simulink model "HalfCar"  (R2020b)
settings: Solver=VariableStepAuto  StartTime=0.0  StopTime=2  MaxStep=0.0001  RelTol=1e-3
values from neighbouring files (symbols this model uses):
  a = 1.233    [main.m]
  Aobs = Aaug-L*Caug    [main.m]
  b = 1.327    [main.m]
  Bobs = [L, Baug]    [main.m]
  Cobs = eye(10)    [main.m]
  Dobs = zeros(10,6)    [main.m]
  kalmanFilter = ss(A_kalman,B_kalman,C_kalman,0)    [main.m]
  Kfeedback = struct('Kf',KFeedb(:,1:8),'P',P)    [main.m]
  KFeedbIntegratore = struct('Kfe',K(:,1:8),'Ki',K(:,9:10),'P',[P,-15-0.1i,-15+.1i ])    [main.m]
  KLQI = struct('KfeLQR',KLQInt(:,1:8),'KiLQR',KLQInt(:,9:10))    [main.m]
  KLQR = struct('KfeLQR',KLQ1(:,1:8))    [main.m]
  varIngressi = 150    [main.m]
  varPhi = 1.0000e-8    (= 1e-08)    [main.m]
  varPhiDot = 1.0000e-7    (= 1e-07)    [main.m]
  varZc = 1.0000e-8    (= 1e-08)    [main.m]
  varZcDot = 1.0000e-7    (= 1e-07)    [main.m]
  veicoloConDisturbi = ss(A,[B,L],C,0)    [main.m]
  vms = convvel(vkmh, 'km/h', 'm/s')    [main.m]
libraries: simulink_extras x18, simulink x2
settings Model: Creator=fadir  LastModifiedBy=fadir

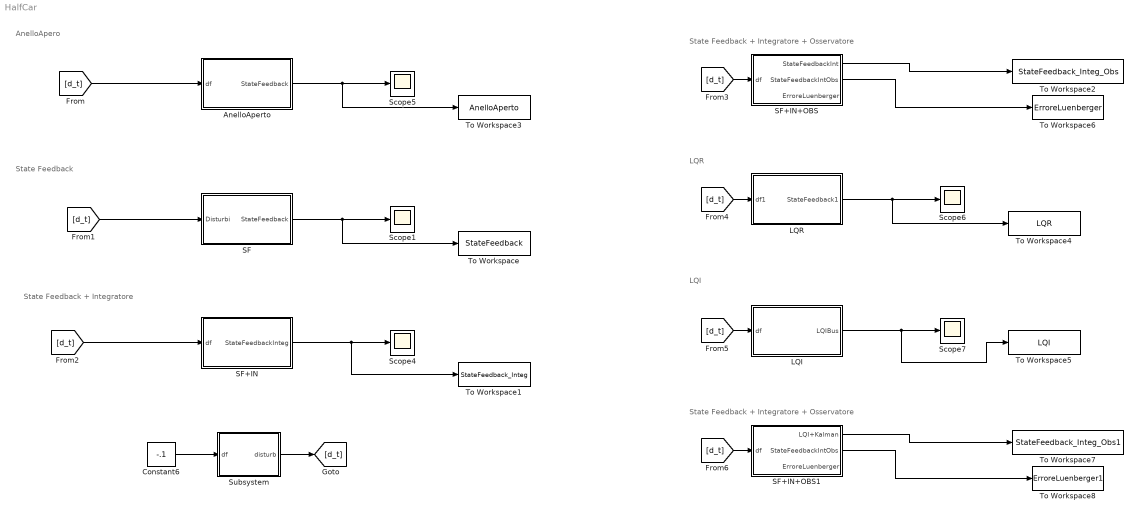
== system HalfCar ==
  note: State Feedback
  note: State Feedback + Integratore + Osservatore
  note: State Feedback + Integratore
  note: AnelloApero
  note: LQR
  note: LQI
  note: State Feedback + Integratore + Osservatore
  AnelloAperto : Subsystem
  Constant6 : Constant  Value=-.1
  LQI : Subsystem
  LQR : Subsystem
  SF : Subsystem
  SF+IN : Subsystem
  SF+IN+OBS : Subsystem
  SF+IN+OBS1 : Subsystem
  Scope{1,4..7} (5 alike) : Scope
  Subsystem : Subsystem
  To Workspace : ToWorkspace  VariableName=StateFeedback  SaveFormat=Timeseries  SampleTime=-1
  To Workspace1 : ToWorkspace  VariableName=StateFeedback_Integ  SaveFormat=Timeseries  SampleTime=-1
  To Workspace2 : ToWorkspace  VariableName=StateFeedback_Integ_Obs  SaveFormat=Timeseries  SampleTime=-1
  To Workspace3 : ToWorkspace  VariableName=AnelloAperto  SaveFormat=Timeseries  SampleTime=-1
  To Workspace4 : ToWorkspace  VariableName=LQR  SaveFormat=Timeseries  SampleTime=-1
  To Workspace5 : ToWorkspace  VariableName=LQI  SaveFormat=Timeseries  SampleTime=-1
  To Workspace6 : ToWorkspace  VariableName=ErroreLuenberger  SaveFormat=Timeseries  SampleTime=-1
  To Workspace7 : ToWorkspace  VariableName=StateFeedback_Integ_Obs1  SaveFormat=Timeseries  SampleTime=-1
  To Workspace8 : ToWorkspace  VariableName=ErroreLuenberger1  SaveFormat=Timeseries  SampleTime=-1
  wires:
  SF/1(StateFeedback) -> To Workspace/1, Scope1/1
  SF+IN+OBS/2(StateFeedbackIntObs) -> To Workspace6/1
  [d_t] -> SF/1(Disturbi)
  [d_t] -> SF+IN+OBS/1(df)
  [d_t] -> SF+IN/1(df)
  SF+IN/1(StateFeedbackInteg) -> To Workspace1/1, Scope4/1
  SF+IN+OBS/1(StateFeedbackInt) -> To Workspace2/1
  AnelloAperto/1(StateFeedback) -> To Workspace3/1, Scope5/1
  [d_t] -> AnelloAperto/1(df)
  [d_t] -> LQR/1(df1)
  LQR/1(StateFeedback1) -> Scope6/1, To Workspace4/1
  LQI/1(LQIBus) -> Scope7/1, To Workspace5/1
  [d_t] -> LQI/1(df)
  Constant6/1 -> Subsystem/1(df)
  Subsystem/1(" disturb") -> [d_t]
  SF+IN+OBS1/1(LQI+Kalman) -> To Workspace7/1
  [d_t] -> SF+IN+OBS1/1(df)
  SF+IN+OBS1/2(StateFeedbackIntObs) -> To Workspace8/1

== system HalfCar/AnelloAperto ==
  df : Inport
  Bus to Vector : BusToVector
  Mux : Mux  Inputs=[2 2]
  State-Space : StateSpace  A=veicoloConDisturbi.A  B=veicoloConDisturbi.B  C=eye(8)  D=zeros(8,4)  InitialCondition=0
  StateFeedbackBus : Subsystem
  StateFeedback : Outport
  wires:
  df/1 -> Bus to Vector/1
  State-Space/1 -> [x_real]  "states"
  Bus to Vector/1 -> Mux/2
  StateFeedbackBus/1(StateFeedback) -> StateFeedback/1
  Mux/1 -> State-Space/1
  [x_real] -> StateFeedbackBus/1(states)

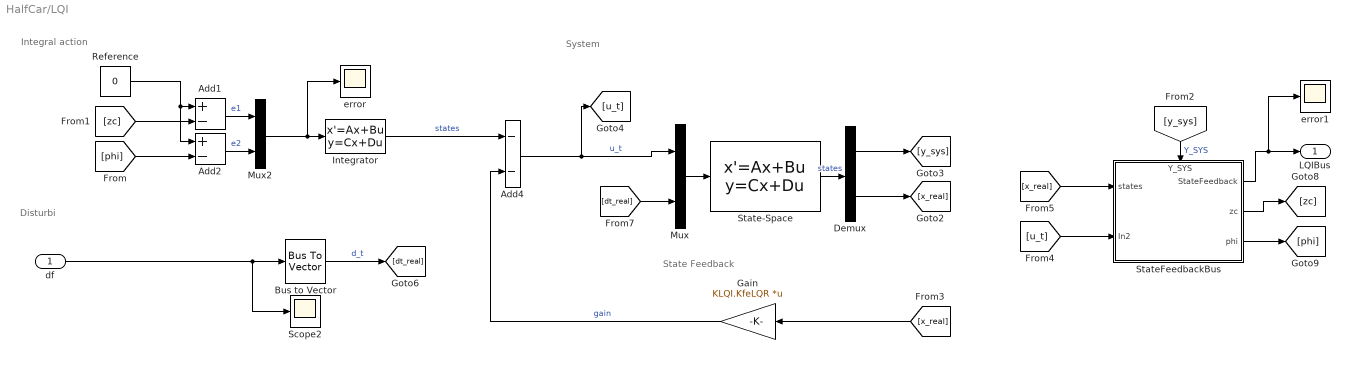
== system HalfCar/LQI ==
  note: System
  note: Integral action
  note: Disturbi
  note: State Feedback
  df : Inport
  Add1 : Sum  Inputs=+-
  Add2 : Sum  Inputs=+-
  Add4 : Sum  Inputs=--
  Bus to Vector : BusToVector
  Demux : Demux  Outputs=[4 8]
  Gain : Gain  Gain=KLQI.KfeLQR  Multiplication=Matrix(K*u)
  Integrator : StateSpace  A=zeros(2,2)  B=KLQI.KiLQR  C=eye(2)  D=zeros(2,2)  InitialCondition=0
  Mux : Mux  Inputs=[2 2]
  Mux2 : Mux  Inputs=2
  Reference : Constant  Value=0
  Scope2 : Scope
  State-Space : StateSpace  A=veicoloConDisturbi.A  B=veicoloConDisturbi.B  C=[veicoloConDisturbi.C;eye(8)]  D=zeros(12,4)  InitialCondition=0
  StateFeedbackBus : Subsystem
      settings: PortSchema="{\"entries\":[{\"content\":{\"sides\":[{\"content\":{\"connectorIds\":[\"In1\",\"In2\"]},\"type\":\"ConnectorPlacement.EquallySpacedRectSide\",\"uuid\":\"f033b987-6b3a-458c-bcac-b7c517520bbe\"},{\"content\":{\"connectorIds\":[\"Out1\",\"Out2\",\"Out3\"],\"side\":\"RIGHT\"},\"type\":\"ConnectorPlacement.EquallySpacedRectSide\",\"uuid\":\"ed7cee92-f0bc-4ba3-a5c5-3396d8293c14\"},{\"content\":{\"connectorIds\":[\"In3\"],\"side\":\"TOP\"},\"type\":\"ConnectorPlacement.EquallySpacedRectSide\",\"uuid\":\"4252f29c-7653-43d7-b93b-010ed3ee46e3\"},{\"content\":{\"connectorIds\":[],\"side\":\"HIDDEN\"},\"type\":\"ConnectorPlacement.EquallySpacedRectSide\",\"uuid\":\"adbffe9e-afd0-46bb-bf47-88a6e7d4714f\"}]},\"type\":\"ConnectorPlacement.EquallySpacedConnector\",\"uuid\":\"76cb68ad-0c01-48a8-b73c-8d6b8ab451c8\"}],\"packageUris\":[\"http://schema.mathworks.com/mf0/Connector/R2020b\"],\"version\":\"1.0\"}"
  error : Scope
  error1 : Scope
  LQIBus : Outport
  wires:
  StateFeedbackBus/2(zc) -> [zc]
  StateFeedbackBus/3(phi) -> [phi]
  StateFeedbackBus/1(" StateFeedback") -> error1/1, LQIBus/1
  [x_real] -> StateFeedbackBus/1(states)
  df/1 -> Bus to Vector/1, Scope2/1
  [zc] -> Add1/2
  [phi] -> Add2/2
  Bus to Vector/1 -> [dt_real]  "d_t"
  Add2/1 -> Mux2/2  "e2"
  Add1/1 -> Mux2/1  "e1"
  Reference/1 -> Add1/1, Add2/1
  Add4/1 -> [u_t], Mux/1  "u_t"
  Integrator/1 -> Add4/1  "states"
  Mux2/1 -> Integrator/1, error/1
  Gain/1 -> Add4/2  "gain"
  Mux/1 -> State-Space/1
  State-Space/1 -> Demux/1  "states"
  Demux/2 -> [x_real]
  [x_real] -> Gain/1
  Demux/1 -> [y_sys]
  [dt_real] -> Mux/2
  [u_t] -> StateFeedbackBus/2(In2)
  [y_sys] -> StateFeedbackBus/3(Y_SYS)  "Y_SYS"

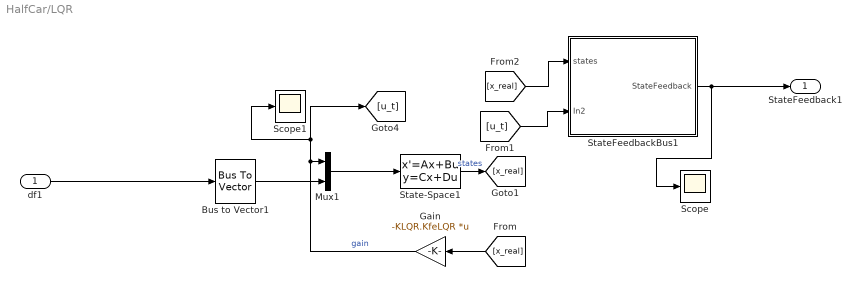
== system HalfCar/LQR ==
  df1 : Inport
  Bus to Vector1 : BusToVector
  Gain : Gain  Gain=-KLQR.KfeLQR  Multiplication=Matrix(K*u)
  Mux1 : Mux  Inputs=[2 2]
  Scope : Scope
  Scope1 : Scope
  State-Space1 : StateSpace  A=veicoloConDisturbi.A  B=veicoloConDisturbi.B  C=eye(8)  D=zeros(8,4)  InitialCondition=0
  StateFeedbackBus1 : Subsystem
  StateFeedback1 : Outport
  wires:
  Mux1/1 -> State-Space1/1
  df1/1 -> Bus to Vector1/1
  State-Space1/1 -> [x_real]  "states"
  Gain/1 -> [u_t], Scope1/1, Mux1/1  "gain"
  [x_real] -> StateFeedbackBus1/1(states)
  [x_real] -> Gain/1
  StateFeedbackBus1/1(StateFeedback) -> Scope/1, StateFeedback1/1
  Bus to Vector1/1 -> Mux1/2
  [u_t] -> StateFeedbackBus1/2(In2)

== system HalfCar/SF ==
  Disturbi : Inport
  Bus to Vector : BusToVector
  Gain : Gain  Gain=-1
  Mux : Mux  Inputs=[2 2]
  RetroazStato : Gain  Gain=Kfeedback.Kf  Multiplication=Matrix(K*u)
  Sistema : StateSpace  A=veicoloConDisturbi.A  B=veicoloConDisturbi.B  C=eye(8)  D=zeros(8,4)  InitialCondition=0
  StateFeedbackBus : Subsystem
  StateFeedback : Outport
  wires:
  RetroazStato/1 -> Gain/1  "gain"
  Disturbi/1 -> Bus to Vector/1
  Sistema/1 -> [x_real]  "states"
  Bus to Vector/1 -> Mux/2
  StateFeedbackBus/1(StateFeedback) -> StateFeedback/1
  Mux/1 -> Sistema/1
  [x_real] -> RetroazStato/1
  [x_real] -> StateFeedbackBus/2(states)
  [u_t] -> StateFeedbackBus/1(u_t)
  Gain/1 -> [u_t], Mux/1

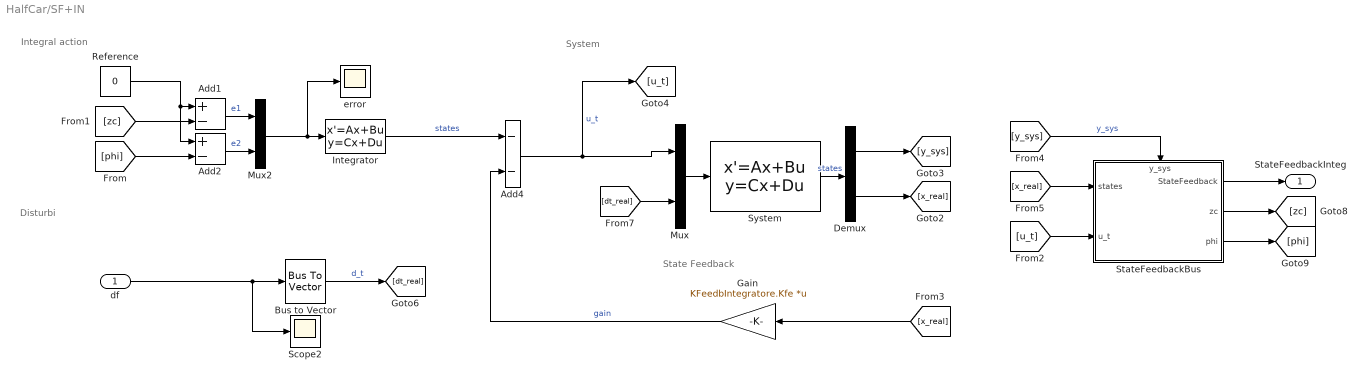
== system HalfCar/SF+IN ==
  note: State Feedback
  note: Disturbi
  note: Integral action
  note: System
  df : Inport
  Add1 : Sum  Inputs=+-
  Add2 : Sum  Inputs=+-
  Add4 : Sum  Inputs=--
  Bus to Vector : BusToVector
  Demux : Demux  Outputs=[4 8]
  Gain : Gain  Gain=KFeedbIntegratore.Kfe  Multiplication=Matrix(K*u)
  Integrator : StateSpace  A=zeros(2,2)  B=KFeedbIntegratore.Ki  C=eye(2)  D=zeros(2,2)  InitialCondition=0
  Mux : Mux  Inputs=[2 2]
  Mux2 : Mux  Inputs=2
  Reference : Constant  Value=0
  Scope2 : Scope
  StateFeedbackBus : Subsystem
      settings: PortSchema="{\"entries\":[{\"content\":{\"sides\":[{\"content\":{\"connectorIds\":[\"In1\",\"In2\"]},\"type\":\"ConnectorPlacement.EquallySpacedRectSide\",\"uuid\":\"7521623e-7228-4753-a009-bff90efec3f5\"},{\"content\":{\"connectorIds\":[\"Out1\",\"Out2\",\"Out3\"],\"side\":\"RIGHT\"},\"type\":\"ConnectorPlacement.EquallySpacedRectSide\",\"uuid\":\"ccf95793-c50d-4e88-afee-999bf5e64e87\"},{\"content\":{\"connectorIds\":[\"In3\"],\"side\":\"TOP\"},\"type\":\"ConnectorPlacement.EquallySpacedRectSide\",\"uuid\":\"63dab736-c292-47ee-a3b5-f2c1b3d06bd7\"},{\"content\":{\"connectorIds\":[],\"side\":\"HIDDEN\"},\"type\":\"ConnectorPlacement.EquallySpacedRectSide\",\"uuid\":\"ac2eb349-1c44-417c-9d28-b58d5fbdbdcb\"}]},\"type\":\"ConnectorPlacement.EquallySpacedConnector\",\"uuid\":\"e4851e5d-b044-4786-a828-79466b73b9fe\"}],\"packageUris\":[\"http://schema.mathworks.com/mf0/Connector/R2020b\"],\"version\":\"1.0\"}"
  System : StateSpace  A=veicoloConDisturbi.A  B=veicoloConDisturbi.B  C=[veicoloConDisturbi.C;eye(8)]  D=zeros(12,4)  InitialCondition=0
  error : Scope
  StateFeedbackInteg : Outport
  wires:
  [dt_real] -> Mux/2
  Demux/1 -> [y_sys]
  [x_real] -> Gain/1
  Demux/2 -> [x_real]
  System/1 -> Demux/1  "states"
  Mux/1 -> System/1
  Gain/1 -> Add4/2  "gain"
  Mux2/1 -> error/1, Integrator/1
  Integrator/1 -> Add4/1  "states"
  Add4/1 -> [u_t], Mux/1  "u_t"
  Reference/1 -> Add2/1, Add1/1
  Add1/1 -> Mux2/1  "e1"
  Add2/1 -> Mux2/2  "e2"
  Bus to Vector/1 -> [dt_real]  "d_t"
  [phi] -> Add2/2
  [zc] -> Add1/2
  df/1 -> Scope2/1, Bus to Vector/1
  [x_real] -> StateFeedbackBus/1(states)
  StateFeedbackBus/1(" StateFeedback") -> StateFeedbackInteg/1
  StateFeedbackBus/3(phi) -> [phi]
  StateFeedbackBus/2(zc) -> [zc]
  [u_t] -> StateFeedbackBus/2(u_t)
  [y_sys] -> StateFeedbackBus/3(y_sys)  "y_sys"

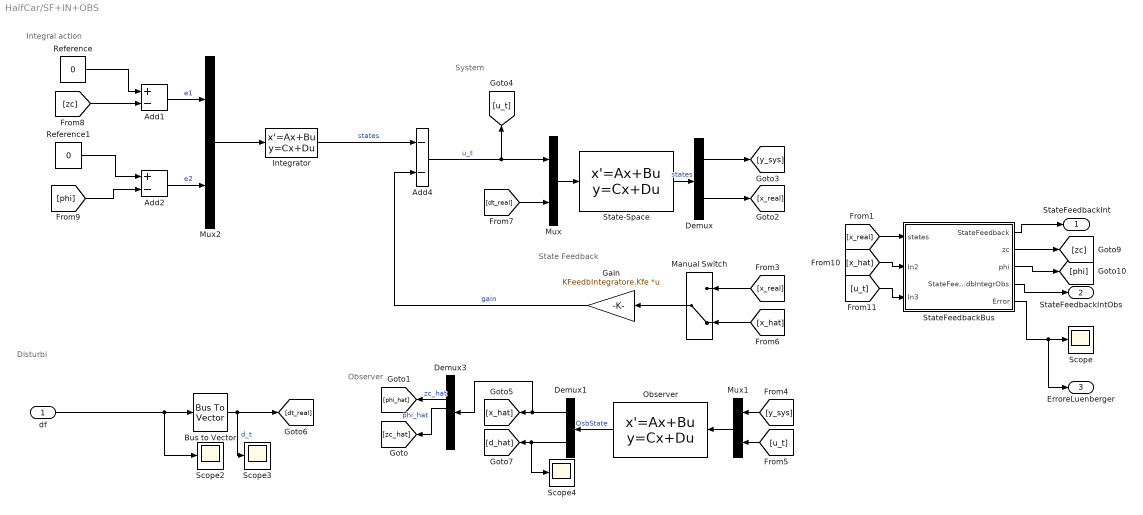
== system HalfCar/SF+IN+OBS ==
  note: System
  note: Observer
  note: Integral action
  note: Disturbi
  note: State Feedback
  df : Inport
  Add1 : Sum  Inputs=+-
  Add2 : Sum  Inputs=+-
  Add4 : Sum  Inputs=--
  Bus to Vector : BusToVector
  Demux : Demux  Outputs=[4 8]
  Demux1 : Demux  Outputs=[8 2]
  Demux3 : Demux  Outputs=8
  Gain : Gain  Gain=KFeedbIntegratore.Kfe  Multiplication=Matrix(K*u)
  Integrator : StateSpace  A=zeros(2,2)  B=KFeedbIntegratore.Ki  C=eye(2)  D=zeros(2,2)  InitialCondition=0
  Manual Switch : ManualSwitch  CurrentSetting=0
  Mux : Mux  Inputs=[2 2]
  Mux1 : Mux  Inputs=2
  Mux2 : Mux  Inputs=2
  Observer : StateSpace  A=Aobs  B=Bobs  C=Cobs  D=Dobs  InitialCondition=[0.121,-0.18,0.4,0.24,-0.3,-0.1,-0.27,0.03,-.04,.003]
  Reference : Constant  Value=0
  Reference1 : Constant  Value=0
  Scope{,2..4} (4 alike) : Scope
  State-Space : StateSpace  A=veicoloConDisturbi.A  B=veicoloConDisturbi.B  C=[veicoloConDisturbi.C;eye(8)]  D=zeros(12,4)  InitialCondition=0
  StateFeedbackBus : Subsystem
  StateFeedbackInt : Outport
  StateFeedbackIntObs : Outport  Port=2
  ErroreLuenberger : Outport  Port=3
  wires:
  df/1 -> Bus to Vector/1, Scope2/1
  Bus to Vector/1 -> Scope3/1, [dt_real]  "d_t"
  Add2/1 -> Mux2/2  "e2"
  Add1/1 -> Mux2/1  "e1"
  Reference/1 -> Add1/1
  Add4/1 -> Mux/1, [u_t]  "u_t"
  Integrator/1 -> Add4/1  "states"
  Mux2/1 -> Integrator/1
  Gain/1 -> Add4/2  "gain"
  Mux/1 -> State-Space/1
  Mux1/1 -> Observer/1
  State-Space/1 -> Demux/1  "states"
  Observer/1 -> Demux1/1  "OsbState"
  Demux1/1 -> Demux3/1, [x_hat]
  Demux1/2 -> Scope4/1, [d_hat]
  Demux/2 -> [x_real]
  Manual Switch/1 -> Gain/1
  [x_real] -> Manual Switch/1
  Demux/1 -> [y_sys]
  [y_sys] -> Mux1/1
  [u_t] -> Mux1/2
  [x_hat] -> Manual Switch/2
  [dt_real] -> Mux/2
  Reference1/1 -> Add2/1
  StateFeedbackBus/3(phi) -> [phi]
  StateFeedbackBus/2(zc) -> [zc]
  [x_real] -> StateFeedbackBus/1(states)
  StateFeedbackBus/1(StateFeedback) -> StateFeedbackInt/1
  StateFeedbackBus/4(StateFeedbIntegrObs) -> StateFeedbackIntObs/1
  [x_hat] -> StateFeedbackBus/2(In2)
  [u_t] -> StateFeedbackBus/3(In3)
  Demux3/3 -> [phi_hat]  "zc_hat"
  Demux3/4 -> [zc_hat]  "phi_hat"
  [zc] -> Add1/2
  [phi] -> Add2/2
  StateFeedbackBus/5("Error ") -> ErroreLuenberger/1, Scope/1

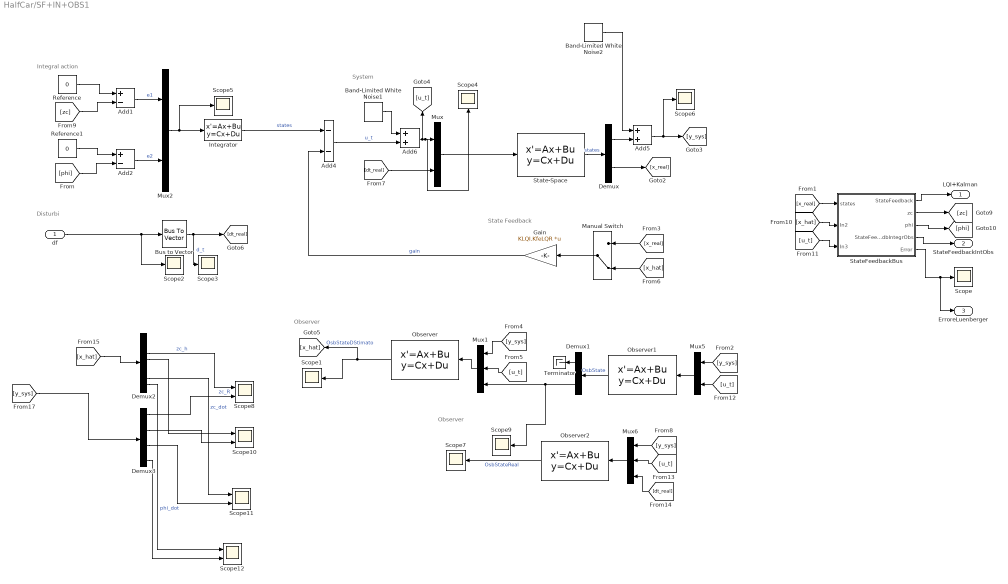
== system HalfCar/SF+IN+OBS1 ==
  note: System
  note: Observer
  note: Integral action
  note: Disturbi
  note: State Feedback
  note: Observer
  df : Inport
  Add1 : Sum  Inputs=+-
  Add2 : Sum  Inputs=+-
  Add4 : Sum  Inputs=--
  Add5 : Sum
  Add6 : Sum
  Band-Limited White Noise1 : simulink/Sources/Band-Limited White Noise  Cov=[varIngressi]  Ts=0.0001  seed=[634913452,25617852]
  Band-Limited White Noise2 : simulink/Sources/Band-Limited White Noise  Cov=[varZc,varPhi,varZcDot,varPhiDot]  Ts=0.0001  seed=[634913452,2315,541416,522131]
  Bus to Vector : BusToVector
  Demux : Demux  Outputs=[4 8]
  Demux1 : Demux  Outputs=[8 2]
  Demux2 : Demux  Outputs=8
  Demux3 : Demux
  Gain : Gain  Gain=KLQI.KfeLQR  Multiplication=Matrix(K*u)
  Integrator : StateSpace  A=zeros(2,2)  B=KLQI.KiLQR  C=eye(2)  D=zeros(2,2)  InitialCondition=0
  Manual Switch : ManualSwitch  CurrentSetting=0
  Mux : Mux  Inputs=[2 2]
  Mux1 : Mux  Inputs=3
  Mux2 : Mux  Inputs=2
  Mux5 : Mux  Inputs=2
  Mux6 : Mux  Inputs=3
  Observer : StateSpace  A=kalmanFilter.A  B=kalmanFilter.B  C=kalmanFilter.C  D=kalmanFilter.D  InitialCondition=zeros(1,8)
  Observer1 : StateSpace  A=Aobs  B=Bobs  C=Cobs  D=Dobs  InitialCondition=[0.121,-0.18,0.4,0.24,-0.3,-0.1,-0.27,0.03,-.04,.003]
  Observer2 : StateSpace  A=kalmanFilter.A  B=kalmanFilter.B  C=kalmanFilter.C  D=kalmanFilter.D  InitialCondition=zeros(1,8)
  Reference : Constant  Value=0
  Reference1 : Constant  Value=0
  Scope{,1..7,9} (9 alike) : Scope
  Scope{8,10..12} (4 alike) : Scope  NumInputPorts=2
  State-Space : StateSpace  A=veicoloConDisturbi.A  B=veicoloConDisturbi.B  C=[veicoloConDisturbi.C;eye(8)]  D=zeros(12,4)  InitialCondition=0
  StateFeedbackBus : Subsystem
  Terminator : Terminator
  LQI+Kalman : Outport
  StateFeedbackIntObs : Outport  Port=2
  ErroreLuenberger : Outport  Port=3
  wires:
  df/1 -> Bus to Vector/1, Scope2/1
  Bus to Vector/1 -> Scope3/1, [dt_real]  "d_t"
  Add2/1 -> Mux2/2  "e2"
  Add1/1 -> Mux2/1  "e1"
  Reference/1 -> Add1/1
  Integrator/1 -> Add4/1  "states"
  Mux2/1 -> Integrator/1, Scope5/1
  Gain/1 -> Add4/2  "gain"
  Mux1/1 -> Observer/1
  State-Space/1 -> Demux/1  "states"
  Observer/1 -> [x_hat], Scope1/1  "OsbStateDStimato"
  Demux/2 -> [x_real]
  Manual Switch/1 -> Gain/1
  [x_real] -> Manual Switch/1
  [y_sys] -> Mux1/1
  [u_t] -> Mux1/2
  [x_hat] -> Manual Switch/2
  Reference1/1 -> Add2/1
  StateFeedbackBus/3(phi) -> [phi]
  StateFeedbackBus/2(zc) -> [zc]
  [x_real] -> StateFeedbackBus/1(states)
  StateFeedbackBus/1(StateFeedback) -> LQI+Kalman/1
  StateFeedbackBus/4(StateFeedbIntegrObs) -> StateFeedbackIntObs/1
  [x_hat] -> StateFeedbackBus/2(In2)
  [u_t] -> StateFeedbackBus/3(In3)
  [zc] -> Add1/2
  [phi] -> Add2/2
  StateFeedbackBus/5("Error ") -> ErroreLuenberger/1, Scope/1
  Mux/1 -> State-Space/1
  Add5/1 -> Scope6/1, [y_sys]
  Demux/1 -> Add5/2
  Demux1/2 -> Scope9/1, Mux1/3
  [y_sys] -> Mux5/1
  Mux5/1 -> Observer1/1
  Observer1/1 -> Demux1/1  "OsbState"
  [u_t] -> Mux5/2
  [u_t] -> Mux6/2
  [y_sys] -> Mux6/1
  Observer2/1 -> Scope7/1  "OsbStateReal"
  Mux6/1 -> Observer2/1
  [dt_real] -> Mux6/3
  Demux1/1 -> Terminator/1
  Add4/1 -> Add6/2  "u_t"
  Add6/1 -> Scope4/1, Mux/1, [u_t]
  [dt_real] -> Mux/2
  Band-Limited White Noise2/1 -> Add5/1
  Band-Limited White Noise1/1 -> Add6/1
  [x_hat] -> Demux2/1
  Demux3/1 -> Scope8/2  "zc_R"
  [y_sys] -> Demux3/1
  Demux2/3 -> Scope8/1  "zc_h"
  Demux3/2 -> Scope10/2
  Demux2/4 -> Scope10/1
  Demux2/7 -> Scope11/1  "zc_dot"
  Demux3/3 -> Scope11/2
  Demux2/8 -> Scope12/1  "phi_dot"
  Demux3/4 -> Scope12/2

== system HalfCar/Subsystem ==
  df : Inport
  Constant1 : Constant  Value=(a+b)
  Constant2 : Constant  Value=1/vms
  Product : Product
  Transfer Fcn1 : TransferFcn  Denominator=[0.05 1]
  Variable Time Delay : VariableTransportDelay  MaximumDelay=10
  Bus Element Out : Outport  PortName=disturb  Element=df
  Bus Element Out1 : Outport  PortName=disturb  Element=dr
  wires:
  Constant2/1 -> Product/2
  Constant1/1 -> Product/1
  df/1 -> Transfer Fcn1/1
  Variable Time Delay/1 -> Bus Element Out1/1  "dr"
  Transfer Fcn1/1 -> Variable Time Delay/1, Bus Element Out/1
  Product/1 -> Variable Time Delay/2

== system HalfCar/AnelloAperto/StateFeedbackBus ==
  states : Inport
  Demux : Demux  Outputs=8
  Radians to Degrees : simulink_extras/Transformations/Radians to Degrees
  Radians to Degrees1 : simulink_extras/Transformations/Radians to Degrees
  Out Bus Element : Outport  PortName=StateFeedback  Element=phi-{[deg]}-{Aperto}
  Out Bus Element1 : Outport  PortName=StateFeedback  Element=phiDot-{[deg]}-{Aperto}
  Out Bus Element2 : Outport  PortName=StateFeedback  Element=zc-{Aperto}
  Out Bus Element3 : Outport  PortName=StateFeedback  Element=zc-{dot}-{Aperto}
  Out Bus Element4 : Outport  PortName=StateFeedback  Element=z1f-{Aperto}
  Out Bus Element5 : Outport  PortName=StateFeedback  Element=z1r-{Aperto}
  Out Bus Element6 : Outport  PortName=StateFeedback  Element=zif-{dot}-{Aperto}
  Out Bus Element7 : Outport  PortName=StateFeedback  Element=zir-{dot}-{Aperto}
  wires:
  Demux/3 -> Out Bus Element2/1  "zc [m]"
  Radians to Degrees1/1 -> Out Bus Element1/1  "phi_dot"
  Demux/4 -> Radians to Degrees/1  "phi"
  Demux/8 -> Radians to Degrees1/1  "phi_dot"
  Radians to Degrees/1 -> Out Bus Element/1  "phi"
  Demux/7 -> Out Bus Element3/1  "zc_dot"
  Demux/1 -> Out Bus Element4/1  "z1f"
  Demux/2 -> Out Bus Element5/1  "z1r"
  Demux/5 -> Out Bus Element6/1  "zif_dot"
  Demux/6 -> Out Bus Element7/1  "zir_dot"
  states/1 -> Demux/1

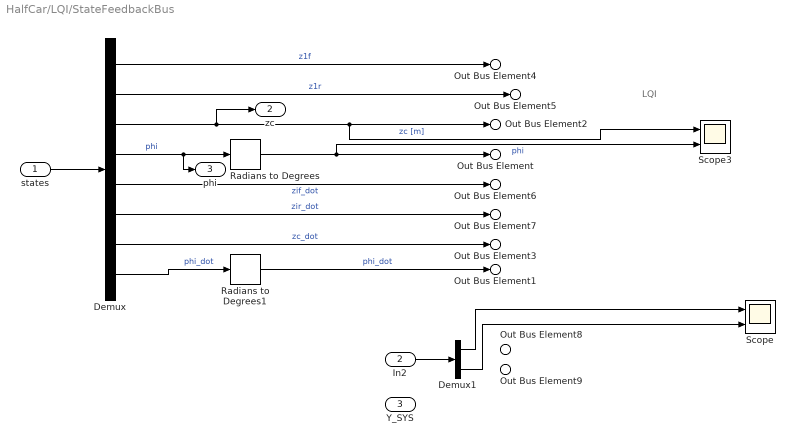
== system HalfCar/LQI/StateFeedbackBus ==
  note: LQI
  states : Inport
  In2 : Inport  Port=2
  Y_SYS : Inport  Port=3
  Demux : Demux  Outputs=8
  Demux1 : Demux  Outputs=2
  Radians to Degrees : simulink_extras/Transformations/Radians to Degrees
  Radians to Degrees1 : simulink_extras/Transformations/Radians to Degrees
  Scope : Scope  NumInputPorts=2
  Scope3 : Scope  NumInputPorts=2
  Out Bus Element : Outport  PortName=StateFeedback  Element=phi-{[deg]}-{LQI}
  Out Bus Element1 : Outport  PortName=StateFeedback  Element=phiDot-{[deg]}-{LQI}
  Out Bus Element2 : Outport  PortName=StateFeedback  Element=zc-{LQI}
  Out Bus Element3 : Outport  PortName=StateFeedback  Element=zc-{dot}-{LQI}
  Out Bus Element4 : Outport  PortName=StateFeedback  Element=z1f-{LQI}
  Out Bus Element5 : Outport  PortName=StateFeedback  Element=z1r-{LQI}
  Out Bus Element6 : Outport  PortName=StateFeedback  Element=zif-{dot}-{LQI}
  Out Bus Element7 : Outport  PortName=StateFeedback  Element=zir-{dot}-{LQI}
  Out Bus Element8 : Outport  PortName=StateFeedback  Element=u_t-{Ant}-{LQI}
  Out Bus Element9 : Outport  PortName=StateFeedback  Element=u_t-{Post}-{LQI}
  zc : Outport  Port=2
  phi : Outport  Port=3
  wires:
  In2/1 -> Demux1/1
  states/1 -> Demux/1
  Demux/6 -> Out Bus Element7/1  "zir_dot"
  Demux/5 -> Out Bus Element6/1  "zif_dot"
  Demux/2 -> Out Bus Element5/1  "z1r"
  Demux/1 -> Out Bus Element4/1  "z1f"
  Demux/7 -> Out Bus Element3/1  "zc_dot"
  Radians to Degrees/1 -> Scope3/2, Out Bus Element/1  "phi"
  Demux/8 -> Radians to Degrees1/1  "phi_dot"
  Demux/4 -> Radians to Degrees/1, phi/1  "phi"
  Radians to Degrees1/1 -> Out Bus Element1/1  "phi_dot"
  Demux/3 -> Scope3/1, Out Bus Element2/1, zc/1  "zc [m]"
  Demux1/1 -> Scope/1
  Demux1/2 -> Scope/2

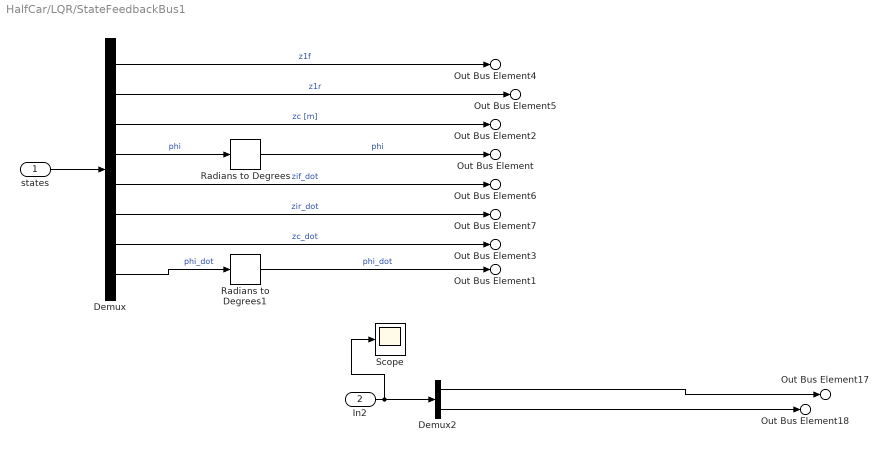
== system HalfCar/LQR/StateFeedbackBus1 ==
  states : Inport
  In2 : Inport  Port=2
  Demux : Demux  Outputs=8
  Demux2 : Demux  Outputs=2
  Radians to Degrees : simulink_extras/Transformations/Radians to Degrees
  Radians to Degrees1 : simulink_extras/Transformations/Radians to Degrees
  Scope : Scope
  Out Bus Element : Outport  PortName=StateFeedback  Element=phi-{[deg]}-{LQR}
  Out Bus Element1 : Outport  PortName=StateFeedback  Element=phiDot-{[deg]}-{LQR}
  Out Bus Element2 : Outport  PortName=StateFeedback  Element=zc-{LQR}
  Out Bus Element3 : Outport  PortName=StateFeedback  Element=zc-{dot}-{LQR}
  Out Bus Element4 : Outport  PortName=StateFeedback  Element=z1f-{LQR}
  Out Bus Element5 : Outport  PortName=StateFeedback  Element=z1r-{LQR}
  Out Bus Element6 : Outport  PortName=StateFeedback  Element=zif-{dot}-{LQR}
  Out Bus Element7 : Outport  PortName=StateFeedback  Element=zir-{dot}-{LQR}
  Out Bus Element17 : Outport  PortName=StateFeedback  Element=u_t-{Ant}-{LQR}
  Out Bus Element18 : Outport  PortName=StateFeedback  Element=u_t-{Post}-{LQR}
  wires:
  Demux/3 -> Out Bus Element2/1  "zc [m]"
  Radians to Degrees1/1 -> Out Bus Element1/1  "phi_dot"
  Demux/4 -> Radians to Degrees/1  "phi"
  Demux/8 -> Radians to Degrees1/1  "phi_dot"
  Radians to Degrees/1 -> Out Bus Element/1  "phi"
  Demux/7 -> Out Bus Element3/1  "zc_dot"
  Demux/1 -> Out Bus Element4/1  "z1f"
  Demux/2 -> Out Bus Element5/1  "z1r"
  Demux/5 -> Out Bus Element6/1  "zif_dot"
  Demux/6 -> Out Bus Element7/1  "zir_dot"
  states/1 -> Demux/1
  In2/1 -> Scope/1, Demux2/1
  Demux2/2 -> Out Bus Element18/1
  Demux2/1 -> Out Bus Element17/1

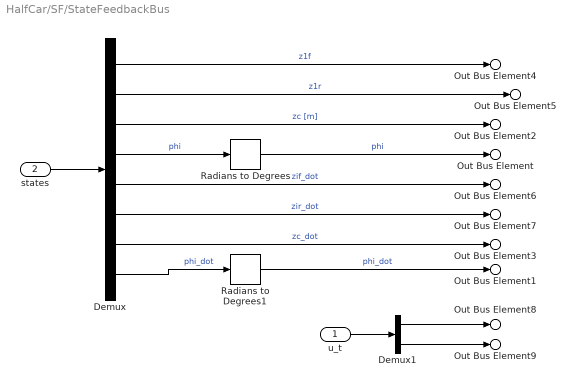
== system HalfCar/SF/StateFeedbackBus ==
  u_t : Inport
  states : Inport  Port=2
  Demux : Demux  Outputs=8
  Demux1 : Demux  Outputs=2
  Radians to Degrees : simulink_extras/Transformations/Radians to Degrees
  Radians to Degrees1 : simulink_extras/Transformations/Radians to Degrees
  Out Bus Element : Outport  PortName=StateFeedback  Element=phi-{[deg]}-{Feed}
  Out Bus Element1 : Outport  PortName=StateFeedback  Element=phiDot-{[deg]}-{Feed}
  Out Bus Element2 : Outport  PortName=StateFeedback  Element=zc-{Feed}
  Out Bus Element3 : Outport  PortName=StateFeedback  Element=zc-{dot}-{Feed}
  Out Bus Element4 : Outport  PortName=StateFeedback  Element=z1f-{Feed}
  Out Bus Element5 : Outport  PortName=StateFeedback  Element=z1r-{Feed}
  Out Bus Element6 : Outport  PortName=StateFeedback  Element=zif-{dot}-{Feed}
  Out Bus Element7 : Outport  PortName=StateFeedback  Element=zir-{dot}-{Feed}
  Out Bus Element8 : Outport  PortName=StateFeedback  Element=u_t-{Ant}-{Feed}
  Out Bus Element9 : Outport  PortName=StateFeedback  Element=u_t-{Post}-{Feed}
  wires:
  Demux/3 -> Out Bus Element2/1  "zc [m]"
  Radians to Degrees1/1 -> Out Bus Element1/1  "phi_dot"
  Demux/4 -> Radians to Degrees/1  "phi"
  Demux/8 -> Radians to Degrees1/1  "phi_dot"
  Radians to Degrees/1 -> Out Bus Element/1  "phi"
  Demux/7 -> Out Bus Element3/1  "zc_dot"
  Demux/1 -> Out Bus Element4/1  "z1f"
  Demux/2 -> Out Bus Element5/1  "z1r"
  Demux/5 -> Out Bus Element6/1  "zif_dot"
  Demux/6 -> Out Bus Element7/1  "zir_dot"
  states/1 -> Demux/1
  u_t/1 -> Demux1/1
  Demux1/1 -> Out Bus Element8/1
  Demux1/2 -> Out Bus Element9/1

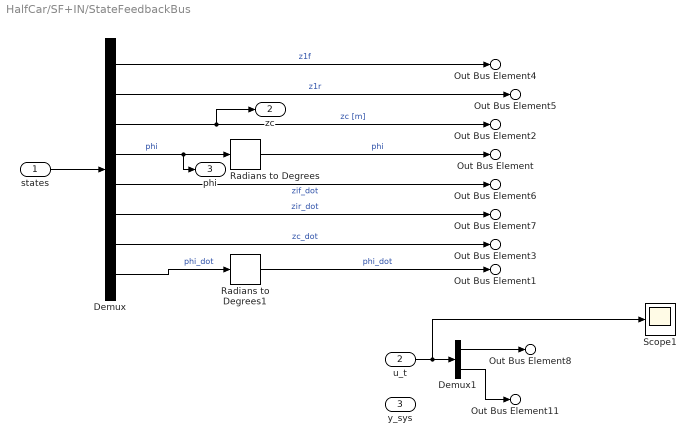
== system HalfCar/SF+IN/StateFeedbackBus ==
  states : Inport
  u_t : Inport  Port=2
  y_sys : Inport  Port=3
  Demux : Demux  Outputs=8
  Demux1 : Demux  Outputs=2
  Radians to Degrees : simulink_extras/Transformations/Radians to Degrees
  Radians to Degrees1 : simulink_extras/Transformations/Radians to Degrees
  Scope1 : Scope
  Out Bus Element : Outport  PortName=StateFeedback  Element=phi-{[deg]}-{FeedInteg}
  Out Bus Element1 : Outport  PortName=StateFeedback  Element=phiDot-{[deg]}-{FeedInteg}
  Out Bus Element2 : Outport  PortName=StateFeedback  Element=zc-{FeedInteg}
  Out Bus Element3 : Outport  PortName=StateFeedback  Element=zc-{dot}-{FeedInteg}
  Out Bus Element4 : Outport  PortName=StateFeedback  Element=z1f-{FeedInteg}
  Out Bus Element5 : Outport  PortName=StateFeedback  Element=z1r-{FeedInteg}
  Out Bus Element6 : Outport  PortName=StateFeedback  Element=zif-{dot}-{FeedInteg}
  Out Bus Element7 : Outport  PortName=StateFeedback  Element=zir-{dot}-{FeedInteg}
  Out Bus Element8 : Outport  PortName=StateFeedback  Element=u_t-{Ant}-{FeedInteg}
  Out Bus Element11 : Outport  PortName=StateFeedback  Element=u_t-{Post}-{FeedInteg}
  zc : Outport  Port=2
  phi : Outport  Port=3
  wires:
  Demux/3 -> zc/1, Out Bus Element2/1  "zc [m]"
  Radians to Degrees1/1 -> Out Bus Element1/1  "phi_dot"
  Demux/4 -> phi/1, Radians to Degrees/1  "phi"
  Demux/8 -> Radians to Degrees1/1  "phi_dot"
  Radians to Degrees/1 -> Out Bus Element/1  "phi"
  Demux/7 -> Out Bus Element3/1  "zc_dot"
  Demux/1 -> Out Bus Element4/1  "z1f"
  Demux/2 -> Out Bus Element5/1  "z1r"
  Demux/5 -> Out Bus Element6/1  "zif_dot"
  Demux/6 -> Out Bus Element7/1  "zir_dot"
  states/1 -> Demux/1
  u_t/1 -> Scope1/1, Demux1/1
  Demux1/1 -> Out Bus Element8/1
  Demux1/2 -> Out Bus Element11/1

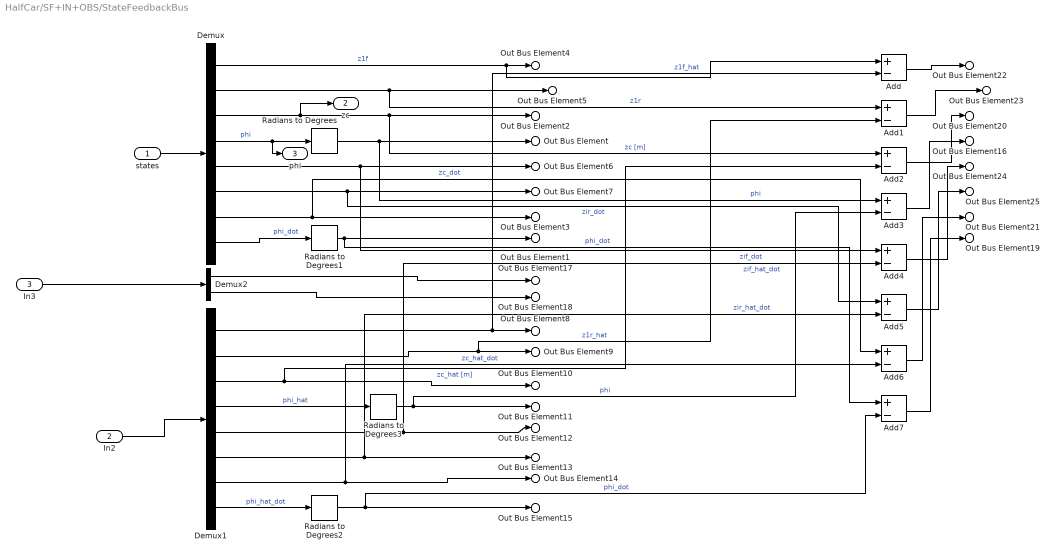
== system HalfCar/SF+IN+OBS/StateFeedbackBus ==
  states : Inport
  In2 : Inport  Port=2
  In3 : Inport  Port=3
  Add{,1..7} (8 alike) : Sum  Inputs=+-
  Demux : Demux  Outputs=8
  Demux1 : Demux  Outputs=8
  Demux2 : Demux  Outputs=2
  Radians to Degrees{,1..3} (4 alike) : simulink_extras/Transformations/Radians to Degrees
  Out Bus Element : Outport  PortName=StateFeedback  Element=phi-{[deg]}-{FeedIntegObs}
  Out Bus Element1 : Outport  PortName=StateFeedback  Element=phiDot-{[deg]}-{FeedIntegObs}
  Out Bus Element2 : Outport  PortName=StateFeedback  Element=zc-{FeedIntegObs}
  Out Bus Element3 : Outport  PortName=StateFeedback  Element=zc-{dot}-{FeedIntegObs}
  Out Bus Element4 : Outport  PortName=StateFeedback  Element=z1f-{FeedIntegObs}
  Out Bus Element5 : Outport  PortName=StateFeedback  Element=z1r-{FeedIntegObs}
  Out Bus Element6 : Outport  PortName=StateFeedback  Element=zif-{dot}-{FeedIntegObs}
  Out Bus Element7 : Outport  PortName=StateFeedback  Element=zir-{dot}-{FeedIntegObs}
  Out Bus Element17 : Outport  PortName=StateFeedback  Element=u_t-{Ant}-{FeedIntegObs}
  Out Bus Element18 : Outport  PortName=StateFeedback  Element=u_t-{Post}-{FeedIntegObs}
  zc : Outport  Port=2
  phi : Outport  Port=3
  Out Bus Element8 : Outport  Port=4  PortName=StateFeedbIntegrObs  Element=z1f-{FeedIntegObs}-{hat}
  Out Bus Element9 : Outport  Port=4  PortName=StateFeedbIntegrObs  Element=z1r-{FeedIntegObs}-{hat}
  Out Bus Element10 : Outport  Port=4  PortName=StateFeedbIntegrObs  Element=zc-{FeedIntegObs}-{hat}
  Out Bus Element11 : Outport  Port=4  PortName=StateFeedbIntegrObs  Element=phi-{[deg]}-{FeedIntegObs}-{hat}
  Out Bus Element12 : Outport  Port=4  PortName=StateFeedbIntegrObs  Element=zif-{dot}-{FeedIntegObs}-{hat}
  Out Bus Element13 : Outport  Port=4  PortName=StateFeedbIntegrObs  Element=zir-{dot}-{FeedIntegObs}-{hat}
  Out Bus Element14 : Outport  Port=4  PortName=StateFeedbIntegrObs  Element=zc-{dot}-{FeedIntegObs}-{hat}
  Out Bus Element15 : Outport  Port=4  PortName=StateFeedbIntegrObs  Element=phiDot-{[deg]}-{FeedIntegObs}-{hat}
  Out Bus Element16 : Outport  Port=5  PortName=Error  Element=phi-{[deg]}-{Error}
  Out Bus Element19 : Outport  Port=5  PortName=Error  Element=phiDot-{[deg]}-{Error}
  Out Bus Element20 : Outport  Port=5  PortName=Error  Element=zc-{Error}
  Out Bus Element21 : Outport  Port=5  PortName=Error  Element=zc-{dot}-{Error}
  Out Bus Element22 : Outport  Port=5  PortName=Error  Element=rz1f-{Error}
  Out Bus Element23 : Outport  Port=5  PortName=Error  Element=z1r-{Error}
  Out Bus Element24 : Outport  Port=5  PortName=Error  Element=zif-{dot}-{Error}
  Out Bus Element25 : Outport  Port=5  PortName=Error  Element=zir-{dot}-{Error}
  wires:
  Demux/3 -> zc/1, Add2/1, Out Bus Element2/1  "zc [m]"
  Radians to Degrees1/1 -> Add7/1, Out Bus Element1/1  "phi_dot"
  Demux/4 -> phi/1, Radians to Degrees/1  "phi"
  Demux/8 -> Radians to Degrees1/1  "phi_dot"
  Radians to Degrees/1 -> Add3/1, Out Bus Element/1  "phi"
  Demux/7 -> Add6/1, Out Bus Element3/1  "zc_dot"
  Demux/1 -> Add/1, Out Bus Element4/1  "z1f"
  Demux/2 -> Add1/1, Out Bus Element5/1  "z1r"
  Demux/5 -> Add4/1, Out Bus Element6/1  "zif_dot"
  Demux/6 -> Add5/1, Out Bus Element7/1  "zir_dot"
  states/1 -> Demux/1
  Demux1/7 -> Add6/2, Out Bus Element14/1  "zc_hat_dot"
  Demux1/8 -> Radians to Degrees2/1  "phi_hat_dot"
  In2/1 -> Demux1/1
  Demux1/2 -> Add1/2, Out Bus Element9/1  "z1r_hat"
  Demux1/3 -> Add2/2, Out Bus Element10/1  "zc_hat [m]"
  Radians to Degrees2/1 -> Add7/2, Out Bus Element15/1  "phi_dot"
  Demux1/6 -> Add5/2, Out Bus Element13/1  "zir_hat_dot"
  Radians to Degrees3/1 -> Add3/2, Out Bus Element11/1  "phi"
  Demux1/1 -> Add/2, Out Bus Element8/1  "z1f_hat"
  Demux1/4 -> Radians to Degrees3/1  "phi_hat"
  Demux1/5 -> Add4/2, Out Bus Element12/1  "zif_hat_dot"
  In3/1 -> Demux2/1
  Demux2/2 -> Out Bus Element18/1
  Demux2/1 -> Out Bus Element17/1
  Add/1 -> Out Bus Element22/1
  Add1/1 -> Out Bus Element23/1
  Add2/1 -> Out Bus Element20/1
  Add3/1 -> Out Bus Element16/1
  Add4/1 -> Out Bus Element24/1
  Add5/1 -> Out Bus Element25/1
  Add6/1 -> Out Bus Element21/1
  Add7/1 -> Out Bus Element19/1

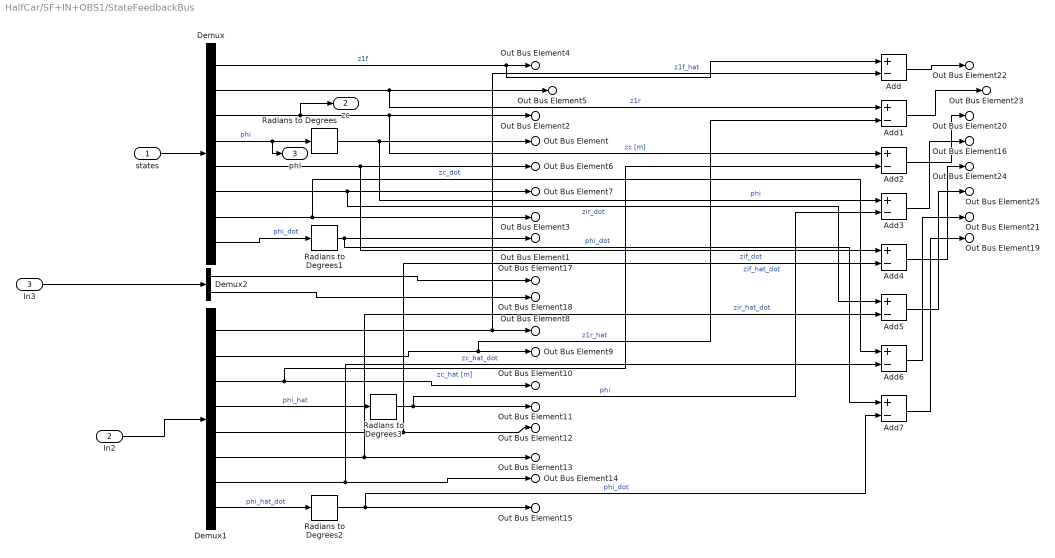
== system HalfCar/SF+IN+OBS1/StateFeedbackBus ==
  states : Inport
  In2 : Inport  Port=2
  In3 : Inport  Port=3
  Add{,1..7} (8 alike) : Sum  Inputs=+-
  Demux : Demux  Outputs=8
  Demux1 : Demux  Outputs=8
  Demux2 : Demux  Outputs=2
  Radians to Degrees{,1..3} (4 alike) : simulink_extras/Transformations/Radians to Degrees
  Out Bus Element : Outport  PortName=StateFeedback  Element=phi-{[deg]}-{FeedIntegObs}
  Out Bus Element1 : Outport  PortName=StateFeedback  Element=phiDot-{[deg]}-{FeedIntegObs}
  Out Bus Element2 : Outport  PortName=StateFeedback  Element=zc-{FeedIntegObs}
  Out Bus Element3 : Outport  PortName=StateFeedback  Element=zc-{dot}-{FeedIntegObs}
  Out Bus Element4 : Outport  PortName=StateFeedback  Element=z1f-{FeedIntegObs}
  Out Bus Element5 : Outport  PortName=StateFeedback  Element=z1r-{FeedIntegObs}
  Out Bus Element6 : Outport  PortName=StateFeedback  Element=zif-{dot}-{FeedIntegObs}
  Out Bus Element7 : Outport  PortName=StateFeedback  Element=zir-{dot}-{FeedIntegObs}
  Out Bus Element17 : Outport  PortName=StateFeedback  Element=u_t-{Ant}-{FeedIntegObs}
  Out Bus Element18 : Outport  PortName=StateFeedback  Element=u_t-{Post}-{FeedIntegObs}
  zc : Outport  Port=2
  phi : Outport  Port=3
  Out Bus Element8 : Outport  Port=4  PortName=StateFeedbIntegrObs  Element=z1f-{FeedIntegObs}-{hat}
  Out Bus Element9 : Outport  Port=4  PortName=StateFeedbIntegrObs  Element=z1r-{FeedIntegObs}-{hat}
  Out Bus Element10 : Outport  Port=4  PortName=StateFeedbIntegrObs  Element=zc-{FeedIntegObs}-{hat}
  Out Bus Element11 : Outport  Port=4  PortName=StateFeedbIntegrObs  Element=phi-{[deg]}-{FeedIntegObs}-{hat}
  Out Bus Element12 : Outport  Port=4  PortName=StateFeedbIntegrObs  Element=zif-{dot}-{FeedIntegObs}-{hat}
  Out Bus Element13 : Outport  Port=4  PortName=StateFeedbIntegrObs  Element=zir-{dot}-{FeedIntegObs}-{hat}
  Out Bus Element14 : Outport  Port=4  PortName=StateFeedbIntegrObs  Element=zc-{dot}-{FeedIntegObs}-{hat}
  Out Bus Element15 : Outport  Port=4  PortName=StateFeedbIntegrObs  Element=phiDot-{[deg]}-{FeedIntegObs}-{hat}
  Out Bus Element16 : Outport  Port=5  PortName=Error  Element=phi-{[deg]}-{Error}
  Out Bus Element19 : Outport  Port=5  PortName=Error  Element=phiDot-{[deg]}-{Error}
  Out Bus Element20 : Outport  Port=5  PortName=Error  Element=zc-{Error}
  Out Bus Element21 : Outport  Port=5  PortName=Error  Element=zc-{dot}-{Error}
  Out Bus Element22 : Outport  Port=5  PortName=Error  Element=rz1f-{Error}
  Out Bus Element23 : Outport  Port=5  PortName=Error  Element=z1r-{Error}
  Out Bus Element24 : Outport  Port=5  PortName=Error  Element=zif-{dot}-{Error}
  Out Bus Element25 : Outport  Port=5  PortName=Error  Element=zir-{dot}-{Error}
  wires:
  Demux/3 -> zc/1, Add2/1, Out Bus Element2/1  "zc [m]"
  Radians to Degrees1/1 -> Add7/1, Out Bus Element1/1  "phi_dot"
  Demux/4 -> phi/1, Radians to Degrees/1  "phi"
  Demux/8 -> Radians to Degrees1/1  "phi_dot"
  Radians to Degrees/1 -> Add3/1, Out Bus Element/1  "phi"
  Demux/7 -> Add6/1, Out Bus Element3/1  "zc_dot"
  Demux/1 -> Add/1, Out Bus Element4/1  "z1f"
  Demux/2 -> Add1/1, Out Bus Element5/1  "z1r"
  Demux/5 -> Add4/1, Out Bus Element6/1  "zif_dot"
  Demux/6 -> Add5/1, Out Bus Element7/1  "zir_dot"
  states/1 -> Demux/1
  Demux1/7 -> Add6/2, Out Bus Element14/1  "zc_hat_dot"
  Demux1/8 -> Radians to Degrees2/1  "phi_hat_dot"
  In2/1 -> Demux1/1
  Demux1/2 -> Add1/2, Out Bus Element9/1  "z1r_hat"
  Demux1/3 -> Add2/2, Out Bus Element10/1  "zc_hat [m]"
  Radians to Degrees2/1 -> Add7/2, Out Bus Element15/1  "phi_dot"
  Demux1/6 -> Add5/2, Out Bus Element13/1  "zir_hat_dot"
  Radians to Degrees3/1 -> Add3/2, Out Bus Element11/1  "phi"
  Demux1/1 -> Add/2, Out Bus Element8/1  "z1f_hat"
  Demux1/4 -> Radians to Degrees3/1  "phi_hat"
  Demux1/5 -> Add4/2, Out Bus Element12/1  "zif_hat_dot"
  In3/1 -> Demux2/1
  Demux2/2 -> Out Bus Element18/1
  Demux2/1 -> Out Bus Element17/1
  Add/1 -> Out Bus Element22/1
  Add1/1 -> Out Bus Element23/1
  Add2/1 -> Out Bus Element20/1
  Add3/1 -> Out Bus Element16/1
  Add4/1 -> Out Bus Element24/1
  Add5/1 -> Out Bus Element25/1
  Add6/1 -> Out Bus Element21/1
  Add7/1 -> Out Bus Element19/1
